simulink model "titop_ol"  (R2018b)
settings: Solver=VariableStepAuto  StartTime=0.0  StopTime=10.0  RelTol=1e-3
values from neighbouring files (symbols this model uses):
  T21 = [cos(theta2) -sin(theta2) 0; sin(theta2) cos(theta2) 0;0 0 1]    [manipulator_titop.m]
undefined symbols (not defined in the file or in its folder): J_payload, m_payload
libraries: cstblocks x2
settings Model: Creator=a.brugnoli  LastModifiedBy=a.brugnoli

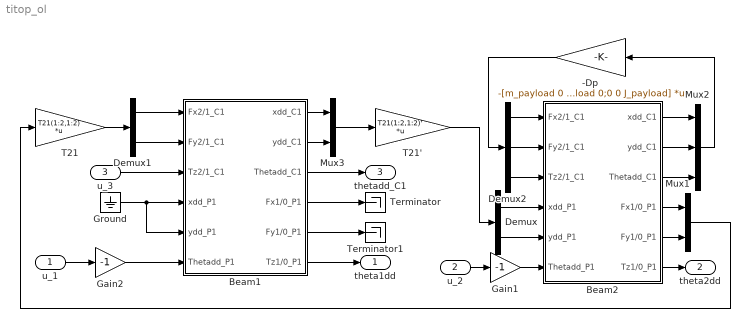
== system titop_ol ==
  u_1 : Inport
  u_2 : Inport  Port=2
  u_3 : Inport  Port=3
  -Dp : Gain  Gain=-[m_payload 0 0;0 m_payload 0;0 0 J_payload]  Multiplication=Matrix(K*u) (u vector)
  Beam1 : Subsystem
  Beam2 : Subsystem
  Demux : Demux  Outputs=2
  Demux1 : Demux  Outputs=2
  Demux2 : Demux  Outputs=3
  Gain1 : Gain  Gain=-1
  Gain2 : Gain  Gain=-1
  Ground : Ground
  Mux1 : Mux  Inputs=2
  Mux2 : Mux  Inputs=3
  Mux3 : Mux  Inputs=2
  T21 : Gain  Gain=T21(1:2,1:2)  Multiplication=Matrix(K*u) (u vector)
  T21' : Gain  Gain=T21(1:2,1:2)'  Multiplication=Matrix(K*u) (u vector)
  Terminator : Terminator
  Terminator1 : Terminator
  theta1dd : Outport
  theta2dd : Outport  Port=2
  thetadd_C1 : Outport  Port=3
  wires:
  Demux1/1 -> Beam1/1(Fx2/1_C1)
  Beam2/1(xdd_C1) -> Mux2/1
  Beam2/6(Tz1/0_P1) -> theta2dd/1
  Beam2/5(Fy1/0_P1) -> Mux1/2
  Beam1/3(Thetadd_C1) -> thetadd_C1/1
  Beam1/5(Fy1/0_P1) -> Terminator1/1
  Beam1/2(ydd_C1) -> Mux3/2
  Beam1/6(Tz1/0_P1) -> theta1dd/1
  Ground/1 -> Beam1/5(ydd_P1), Beam1/4(xdd_P1)
  T21'/1 -> Demux/1
  Mux1/1 -> T21/1
  Demux2/2 -> Beam2/2(Fy2/1_C1)
  -Dp/1 -> Demux2/1
  Beam1/4(Fx1/0_P1) -> Terminator/1
  Demux2/1 -> Beam2/1(Fx2/1_C1)
  Mux2/1 -> -Dp/1
  Beam2/3(Thetadd_C1) -> Mux2/3
  Demux1/2 -> Beam1/2(Fy2/1_C1)
  Beam2/2(ydd_C1) -> Mux2/2
  Demux/2 -> Beam2/5(ydd_P1)
  Demux/1 -> Beam2/4(xdd_P1)
  Demux2/3 -> Beam2/3(Tz2/1_C1)
  Beam2/4(Fx1/0_P1) -> Mux1/1
  T21/1 -> Demux1/1
  Mux3/1 -> T21'/1
  Beam1/1(xdd_C1) -> Mux3/1
  u_1/1 -> Gain2/1
  u_2/1 -> Gain1/1
  Gain2/1 -> Beam1/6("Thetadd_P1 ")
  Gain1/1 -> Beam2/6("Thetadd_P1 ")
  u_3/1 -> Beam1/3(Tz2/1_C1)

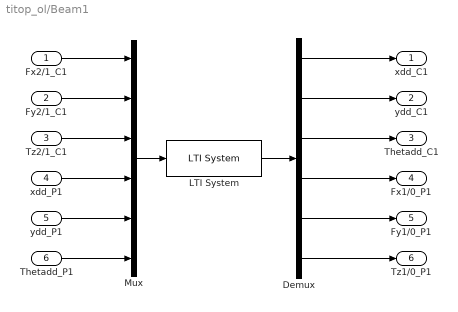
== system titop_ol/Beam1 ==
  Fx2/1_C1 : Inport
  Fy2/1_C1 : Inport  Port=2
  Tz2/1_C1 : Inport  Port=3
  xdd_P1 : Inport  Port=4
  ydd_P1 : Inport  Port=5
  "Thetadd_P1 " : Inport  Port=6
  Demux : Demux  Outputs=6
  LTI System : cstblocks/LTI System  sys=Maug1  IC=[]
  Mux : Mux  Inputs=6
  xdd_C1 : Outport
  ydd_C1 : Outport  Port=2
  Thetadd_C1 : Outport  Port=3
  Fx1/0_P1 : Outport  Port=4
  Fy1/0_P1 : Outport  Port=5
  Tz1/0_P1 : Outport  Port=6
  wires:
  Fx2/1_C1/1 -> Mux/1
  Fy2/1_C1/1 -> Mux/2
  Tz2/1_C1/1 -> Mux/3
  xdd_P1/1 -> Mux/4
  "Thetadd_P1 "/1 -> Mux/6
  ydd_P1/1 -> Mux/5
  Mux/1 -> LTI System/1
  LTI System/1 -> Demux/1
  Demux/1 -> xdd_C1/1
  Demux/2 -> ydd_C1/1
  Demux/3 -> Thetadd_C1/1
  Demux/4 -> Fx1/0_P1/1
  Demux/5 -> Fy1/0_P1/1
  Demux/6 -> Tz1/0_P1/1

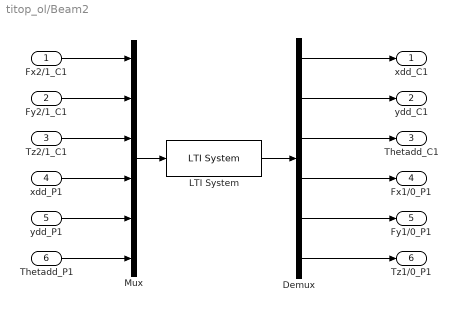
== system titop_ol/Beam2 ==
  Fx2/1_C1 : Inport
  Fy2/1_C1 : Inport  Port=2
  Tz2/1_C1 : Inport  Port=3
  xdd_P1 : Inport  Port=4
  ydd_P1 : Inport  Port=5
  "Thetadd_P1 " : Inport  Port=6
  Demux : Demux  Outputs=6
  LTI System : cstblocks/LTI System  sys=Maug2  IC=[]
  Mux : Mux  Inputs=6
  xdd_C1 : Outport
  ydd_C1 : Outport  Port=2
  Thetadd_C1 : Outport  Port=3
  Fx1/0_P1 : Outport  Port=4
  Fy1/0_P1 : Outport  Port=5
  Tz1/0_P1 : Outport  Port=6
  wires:
  Demux/4 -> Fx1/0_P1/1
  Demux/1 -> xdd_C1/1
  ydd_P1/1 -> Mux/5
  Mux/1 -> LTI System/1
  LTI System/1 -> Demux/1
  Demux/3 -> Thetadd_C1/1
  Fx2/1_C1/1 -> Mux/1
  Demux/2 -> ydd_C1/1
  Demux/5 -> Fy1/0_P1/1
  xdd_P1/1 -> Mux/4
  Demux/6 -> Tz1/0_P1/1
  Fy2/1_C1/1 -> Mux/2
  "Thetadd_P1 "/1 -> Mux/6
  Tz2/1_C1/1 -> Mux/3
